simulink model "Tarefa02"  (R2016a)
settings: Solver=VariableStepAuto  StartTime=0.0  StopTime=1.6e-3  RelTol=1e-3
libraries: dspxfrm3 x6, dspfdesign x3
settings Model: Creator=pedro  LastModifiedBy=pedro

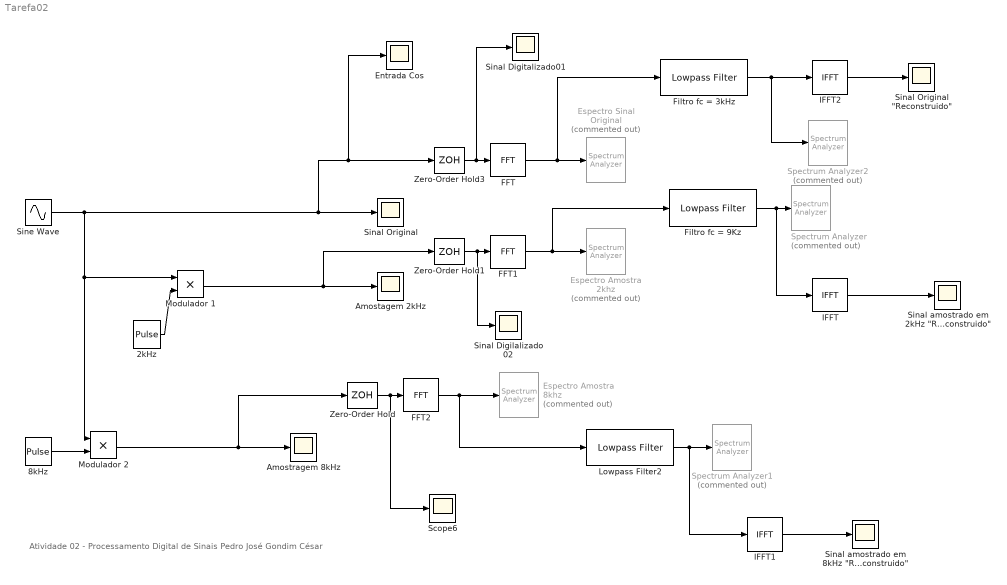
== system Tarefa02 ==
  note: Atividade 02 - Processamento Digital de Sinais
      | Pedro José Gondim César
  "\tModulador 1" : Product
  2kHz : DiscretePulseGenerator  PulseType=Time based  Period=5e-4  PulseWidth=10
  8kHz : DiscretePulseGenerator  PulseType=Time based  Period=1.25e-4/2  PulseWidth=5
  Amostagem 2kHz : Scope
  Amostragem 8kHz : Scope
  Entrada Cos : Scope
  Espectro Amostra 2khz : SpectrumAnalyzer  Commented=on
  Espectro Amostra 8khz : SpectrumAnalyzer  Commented=on
  Espectro Sinal Original : SpectrumAnalyzer  Commented=on
  FFT : dspxfrm3/FFT  FFTImplementation=Auto  CompMethod=Table lookup  TableOpt=NEW  TableOptActive=Speed  BitRevOrder=off  Normalize=off  InheritFFTLength=on  FFTLength=64  WrapInput=on  roundingMode=Floor  overflowMode=off  firstCoeffDataTypeStr=Inherit: Same word length as input  firstCoeffLastDataTypeStr=Inherit: Same word length as input  outputMin=[]  outputMax=[]
  FFT1 : dspxfrm3/FFT  FFTImplementation=Auto  CompMethod=Table lookup  TableOpt=NEW  TableOptActive=Speed  BitRevOrder=off  Normalize=off  InheritFFTLength=on  FFTLength=64  WrapInput=on  roundingMode=Floor  overflowMode=off  firstCoeffDataTypeStr=Inherit: Same word length as input  firstCoeffLastDataTypeStr=Inherit: Same word length as input  outputMin=[]  outputMax=[]
  FFT2 : dspxfrm3/FFT  FFTImplementation=Auto  CompMethod=Table lookup  TableOpt=NEW  TableOptActive=Speed  BitRevOrder=off  Normalize=off  InheritFFTLength=on  FFTLength=64  WrapInput=on  roundingMode=Floor  overflowMode=off  firstCoeffDataTypeStr=Inherit: Same word length as input  firstCoeffLastDataTypeStr=Inherit: Same word length as input  outputMin=[]  outputMax=[]
  Filtro fc = 3kHz : dspfdesign/Lowpass Filter  FilterType=FIR  DesignForMinimumOrder=on  FilterOrder=50  PassbandFrequency=8e3  StopbandFrequency=9e3  PassbandRipple=0.1  StopbandAttenuation=80  InheritSampleRate=off  SampleRate=44100  roundingMode=Floor  coeffsDataTypeStr=fixdt(1,16)  SimulateUsing=Interpreted execution
  Filtro fc = 9Kz : dspfdesign/Lowpass Filter  FilterType=FIR  DesignForMinimumOrder=on  FilterOrder=50  PassbandFrequency=2e3  StopbandFrequency=3e3  PassbandRipple=0.1  StopbandAttenuation=80  InheritSampleRate=off  SampleRate=44100  roundingMode=Floor  coeffsDataTypeStr=fixdt(1,16)  SimulateUsing=Interpreted execution
  IFFT : dspxfrm3/IFFT  FFTImplementation=Auto  CompMethod=Table lookup  TableOpt=NEW  TableOptActive=Speed  BitRevOrder=off  cs_in=off  Normalize=on  InheritFFTLength=on  FFTLength=64  WrapInput=on  mode=Complex  outSamplingMode=Sample based  roundingMode=Floor  overflowMode=off  firstCoeffDataTypeStr=Inherit: Same word length as input  firstCoeffLastDataTypeStr=Inherit: Same word length as input  outputMin=[]  outputMax=[]
  IFFT1 : dspxfrm3/IFFT  FFTImplementation=Auto  CompMethod=Table lookup  TableOpt=NEW  TableOptActive=Speed  BitRevOrder=off  cs_in=off  Normalize=on  InheritFFTLength=on  FFTLength=64  WrapInput=on  mode=Complex  outSamplingMode=Sample based  roundingMode=Floor  overflowMode=off  firstCoeffDataTypeStr=Inherit: Same word length as input  firstCoeffLastDataTypeStr=Inherit: Same word length as input  outputMin=[]  outputMax=[]
  IFFT2 : dspxfrm3/IFFT  FFTImplementation=Auto  CompMethod=Table lookup  TableOpt=NEW  TableOptActive=Speed  BitRevOrder=off  cs_in=off  Normalize=on  InheritFFTLength=on  FFTLength=64  WrapInput=on  mode=Complex  outSamplingMode=Sample based  roundingMode=Floor  overflowMode=off  firstCoeffDataTypeStr=Inherit: Same word length as input  firstCoeffLastDataTypeStr=Inherit: Same word length as input  outputMin=[]  outputMax=[]
  Lowpass Filter2 : dspfdesign/Lowpass Filter  FilterType=FIR  DesignForMinimumOrder=on  FilterOrder=50  PassbandFrequency=8e3  StopbandFrequency=9e3  PassbandRipple=0.1  StopbandAttenuation=80  InheritSampleRate=off  SampleRate=44100  roundingMode=Floor  coeffsDataTypeStr=fixdt(1,16)  SimulateUsing=Interpreted execution
  Modulador 2 : Product
  Scope6 : Scope
  Sinal Digilalizado 02 : Scope
  Sinal Digitalizado01 : Scope
  Sinal Original : Scope
  "Sinal Original \"Reconstruido\"" : Scope
  "Sinal amostrado em 2kHz \"Reconstruido\"" : Scope
  "Sinal amostrado em 8kHz \"Reconstruido\"" : Scope
  Sine Wave : Sin  Frequency=2*pi*7*10^3  SampleTime=0
  Spectrum Analyzer : SpectrumAnalyzer  Commented=on
  Spectrum Analyzer1 : SpectrumAnalyzer  Commented=on
  Spectrum Analyzer2 : SpectrumAnalyzer  Commented=on
  Zero-Order Hold : ZeroOrderHold  SampleTime=1e-6
  Zero-Order Hold1 : ZeroOrderHold  SampleTime=1e-6
  Zero-Order Hold3 : ZeroOrderHold  SampleTime=1e-6
  wires:
  2kHz/1 -> "\tModulador 1"/2
  8kHz/1 -> Modulador 2/2
  "\tModulador 1"/1 -> Zero-Order Hold1/1, Amostagem 2kHz/1
  Modulador 2/1 -> Amostragem 8kHz/1, Zero-Order Hold/1
  FFT2/1 -> Lowpass Filter2/1, Espectro Amostra 8khz/1
  FFT1/1 -> Filtro fc = 9Kz/1, Espectro Amostra 2khz/1
  FFT/1 -> Filtro fc = 3kHz/1, Espectro Sinal Original/1
  Zero-Order Hold/1 -> Scope6/1, FFT2/1
  Zero-Order Hold1/1 -> Sinal Digilalizado 02/1, FFT1/1
  Zero-Order Hold3/1 -> Sinal Digitalizado01/1, FFT/1
  Lowpass Filter2/1 -> IFFT1/1, Spectrum Analyzer1/1
  Filtro fc = 9Kz/1 -> IFFT/1, Spectrum Analyzer/1
  IFFT/1 -> "Sinal amostrado em 2kHz \"Reconstruido\""/1
  IFFT1/1 -> "Sinal amostrado em 8kHz \"Reconstruido\""/1
  Filtro fc = 3kHz/1 -> Spectrum Analyzer2/1, IFFT2/1
  IFFT2/1 -> "Sinal Original \"Reconstruido\""/1
  Sine Wave/1 -> Modulador 2/1, "\tModulador 1"/1, Entrada Cos/1, Zero-Order Hold3/1, Sinal Original/1
